simulink model "Final_Project_Part_4_LVLH_kinematics_Template"  (R2022a)
settings: Solver=ode45  StartTime=0.0  StopTime=tspan  RelTol=1e-8  AbsTol=1e-8
model workspace (MATLAB code in the model file):
  | mu = 398601; % km
  | Re = 6378.137; %km
values from neighbouring files (symbols this model uses):
  J = I/12 - m * rx * rx    [aero421_finalProject.m]    (also in aero421_finalProject_D.m)
undefined symbols (not defined in the file or in its folder): E_b_ECI_0, E_b_LVLH_0, q_b_ECI_0, q_b_LVLH_0, r_ECI_0, T_c, v_ECI_0, w_b_ECI_0
settings Model: Creator=emehiel  LastModifiedBy=emehiel
settings SolverCC: AlgebraicLoopSolver=TrustRegion
settings DebuggingCC: UnconnectedInputMsg=warning  UnconnectedOutputMsg=warning  UnconnectedLineMsg=warning  SFMachineParentedDataDiag=warning

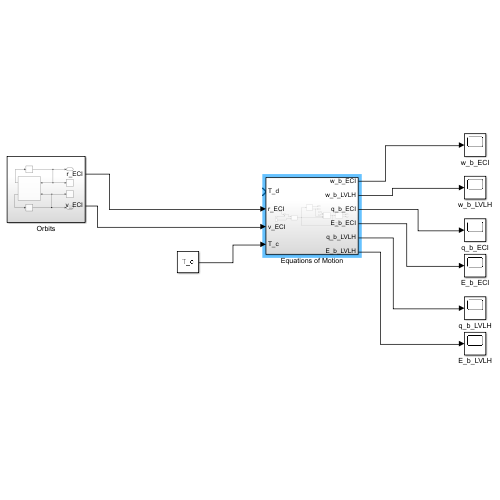
[thumbnail: Simulink's stored preview of the top-level diagram]
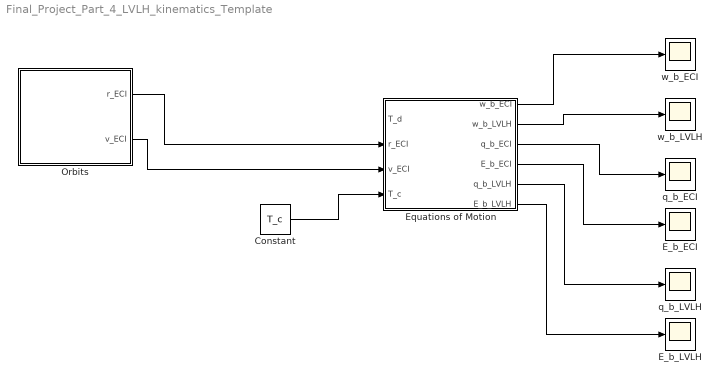
== system Final_Project_Part_4_LVLH_kinematics_Template ==
  Constant : Constant  Value=T_c
  E_b_ECI : Scope
  E_b_LVLH : Scope
  Equations of Motion : Subsystem
  Orbits : Subsystem
  q_b_ECI : Scope
  q_b_LVLH : Scope
  w_b_ECI : Scope
  w_b_LVLH : Scope
  wires:
  Orbits/1(r_ECI) -> Equations of Motion/2(r_ECI)
  Equations of Motion/3(q_b_ECI) -> q_b_ECI/1
  Equations of Motion/1(w_b_ECI) -> w_b_ECI/1
  Equations of Motion/4(E_b_ECI) -> E_b_ECI/1
  Equations of Motion/2(w_b_LVLH) -> w_b_LVLH/1
  Equations of Motion/5(q_b_LVLH) -> q_b_LVLH/1
  Equations of Motion/6(E_b_LVLH) -> E_b_LVLH/1
  Orbits/2(v_ECI) -> Equations of Motion/3(v_ECI)
  Constant/1 -> Equations of Motion/4(T_c)

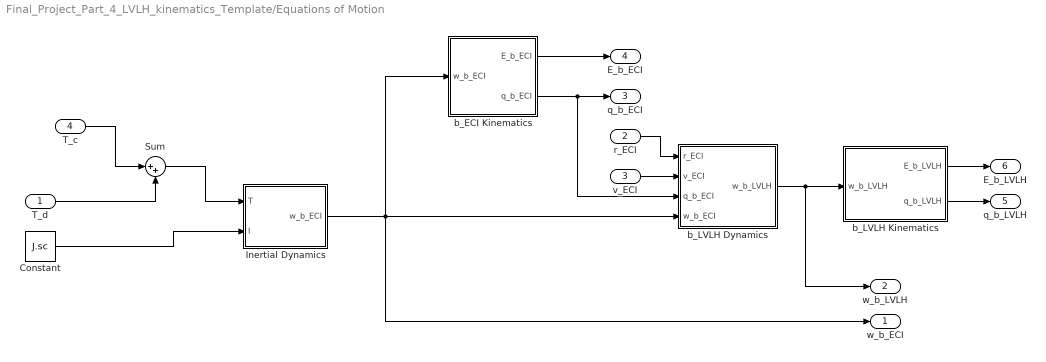
== system Final_Project_Part_4_LVLH_kinematics_Template/Equations of Motion ==
  T_d : Inport
  r_ECI : Inport  Port=2
  v_ECI : Inport  Port=3
  T_c : Inport  Port=4
  Constant : Constant  Value=J.sc
  Inertial Dynamics : Subsystem
  Sum : Sum  Inputs=|++
  b_ECI Kinematics : Subsystem
  b_LVLH Dynamics : Subsystem
  b_LVLH Kinematics : Subsystem
  w_b_ECI : Outport  VectorParamsAs1DForOutWhenUnconnected=off
  w_b_LVLH : Outport  Port=2  PortDimensions=[3 1]  VectorParamsAs1DForOutWhenUnconnected=off
  q_b_ECI : Outport  Port=3  PortDimensions=[4 1]  VectorParamsAs1DForOutWhenUnconnected=off
  E_b_ECI : Outport  Port=4  PortDimensions=[3 1]  VectorParamsAs1DForOutWhenUnconnected=off
  q_b_LVLH : Outport  Port=5  PortDimensions=[4 1]  VectorParamsAs1DForOutWhenUnconnected=off
  E_b_LVLH : Outport  Port=6  PortDimensions=[3 1]  VectorParamsAs1DForOutWhenUnconnected=off
  wires:
  b_ECI Kinematics/1(E_b_ECI) -> E_b_ECI/1
  Constant/1 -> Inertial Dynamics/2(I)
  b_LVLH Kinematics/1(E_b_LVLH) -> E_b_LVLH/1
  Inertial Dynamics/1(w_b_ECI) -> w_b_ECI/1, b_ECI Kinematics/1(w_b_ECI), b_LVLH Dynamics/4(w_b_ECI)
  b_ECI Kinematics/2(q_b_ECI) -> b_LVLH Dynamics/3(q_b_ECI), q_b_ECI/1
  b_LVLH Kinematics/2(q_b_LVLH) -> q_b_LVLH/1
  r_ECI/1 -> b_LVLH Dynamics/1("r_ECI ")
  v_ECI/1 -> b_LVLH Dynamics/2(v_ECI)
  b_LVLH Dynamics/1(w_b_LVLH) -> w_b_LVLH/1, b_LVLH Kinematics/1(w_b_LVLH)
  T_d/1 -> Sum/2
  T_c/1 -> Sum/1
  Sum/1 -> Inertial Dynamics/1(T)

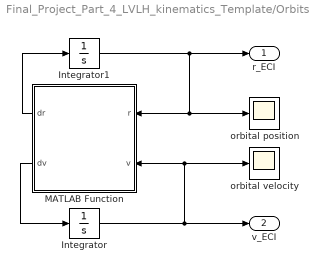
== system Final_Project_Part_4_LVLH_kinematics_Template/Orbits ==
  Integrator : Integrator  InitialCondition=v_ECI_0
  Integrator1 : Integrator  InitialCondition=r_ECI_0
  MATLAB Function : MATLAB Function  TreatAsAtomicUnit=on
  orbital position : Scope
  orbital velocity : Scope
  r_ECI : Outport  VectorParamsAs1DForOutWhenUnconnected=off
  v_ECI : Outport  Port=2  VectorParamsAs1DForOutWhenUnconnected=off
  wires:
  Integrator/1 -> orbital velocity/1, MATLAB Function/2(v), v_ECI/1
  Integrator1/1 -> orbital position/1, MATLAB Function/1(r), r_ECI/1
  MATLAB Function/1(dr) -> Integrator1/1
  MATLAB Function/2(dv) -> Integrator/1

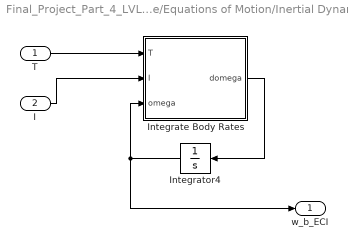
== system Final_Project_Part_4_LVLH_kinematics_Template/Equations of Motion/Inertial Dynamics ==
  T : Inport
  I : Inport  Port=2
  Integrate Body Rates : MATLAB Function  TreatAsAtomicUnit=on
  Integrator4 : Integrator  InitialCondition=w_b_ECI_0
  w_b_ECI : Outport  VectorParamsAs1DForOutWhenUnconnected=off
  wires:
  Integrate Body Rates/1(domega) -> Integrator4/1
  I/1 -> Integrate Body Rates/2(I)
  T/1 -> Integrate Body Rates/1(T)
  Integrator4/1 -> w_b_ECI/1, Integrate Body Rates/3(omega)

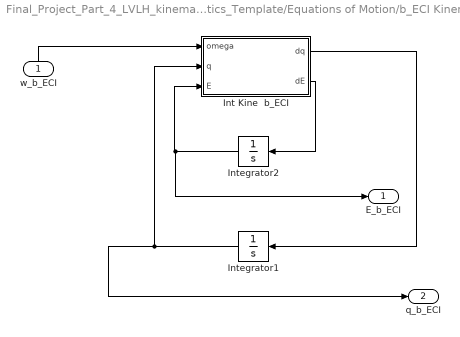
== system Final_Project_Part_4_LVLH_kinematics_Template/Equations of Motion/b_ECI Kinematics ==
  w_b_ECI : Inport
  Int Kine  b_ECI : MATLAB Function  TreatAsAtomicUnit=on
  Integrator1 : Integrator  InitialCondition=q_b_ECI_0
  Integrator2 : Integrator  InitialCondition=E_b_ECI_0
  E_b_ECI : Outport  PortDimensions=[3 1]  VectorParamsAs1DForOutWhenUnconnected=off
  q_b_ECI : Outport  Port=2  PortDimensions=[4 1]  VectorParamsAs1DForOutWhenUnconnected=off
  wires:
  w_b_ECI/1 -> Int Kine  b_ECI/1(omega)
  Int Kine  b_ECI/1(dq) -> Integrator1/1
  Int Kine  b_ECI/2(dE) -> Integrator2/1
  Integrator1/1 -> q_b_ECI/1, Int Kine  b_ECI/2(q)
  Integrator2/1 -> E_b_ECI/1, Int Kine  b_ECI/3(E)

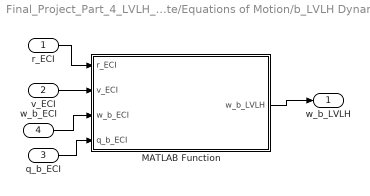
== system Final_Project_Part_4_LVLH_kinematics_Template/Equations of Motion/b_LVLH Dynamics ==
  "r_ECI " : Inport
  v_ECI : Inport  Port=2
  q_b_ECI : Inport  Port=3
  w_b_ECI : Inport  Port=4
  MATLAB Function : MATLAB Function  TreatAsAtomicUnit=on
  w_b_LVLH : Outport  VectorParamsAs1DForOutWhenUnconnected=off
  wires:
  MATLAB Function/1(w_b_LVLH) -> w_b_LVLH/1
  "r_ECI "/1 -> MATLAB Function/1(r_ECI)
  v_ECI/1 -> MATLAB Function/2(v_ECI)
  q_b_ECI/1 -> MATLAB Function/4(q_b_ECI)
  w_b_ECI/1 -> MATLAB Function/3(w_b_ECI)

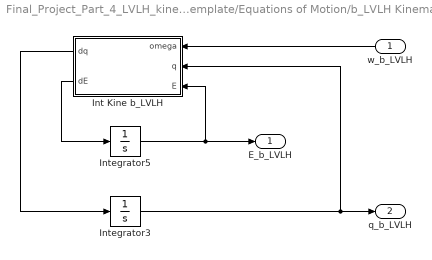
== system Final_Project_Part_4_LVLH_kinematics_Template/Equations of Motion/b_LVLH Kinematics ==
  w_b_LVLH : Inport
  Int Kine b_LVLH : MATLAB Function  TreatAsAtomicUnit=on
  Integrator3 : Integrator  InitialCondition=q_b_LVLH_0
  Integrator5 : Integrator  InitialCondition=E_b_LVLH_0
  E_b_LVLH : Outport  PortDimensions=[3 1]  VectorParamsAs1DForOutWhenUnconnected=off
  q_b_LVLH : Outport  Port=2  VectorParamsAs1DForOutWhenUnconnected=off
  wires:
  Int Kine b_LVLH/1(dq) -> Integrator3/1
  Integrator3/1 -> Int Kine b_LVLH/2(q), q_b_LVLH/1
  Int Kine b_LVLH/2(dE) -> Integrator5/1
  Integrator5/1 -> E_b_LVLH/1, Int Kine b_LVLH/3(E)
  w_b_LVLH/1 -> Int Kine b_LVLH/1(omega)

== matlab function Final_Project_Part_4_LVLH_kinematics_Template/Equations of Motion/Inertial Dynamics/Integrate Body Rates ==
  data: T input; I input; omega input; domega output
function domega = dynamics(T, I, omega)
%#codegen

domega = I\(T - cross(omega, I*omega));

== matlab function Final_Project_Part_4_LVLH_kinematics_Template/Equations of Motion/b_ECI Kinematics/Int Kine  b_ECI ==
  data: omega input; q input; dq output; E input; dE output
function [dq,dE] = kinematics(omega, q, E)
%#codegen

% unpack quaternion

epsilon = q(1:3,1);
eta = q(4,1);

depsilon = 1/2*(eta*eye(3) + vect2cross(epsilon))*omega;
deta = -1/2*epsilon'*omega;

dq = [depsilon; deta];

LBI = 1/cos(E(2))*[cos(E(2)) sin(E(1))*sin(E(2))  cos(E(1))*sin(E(2));
                   0         cos(E(1))*cos(E(2)) -sin(E(1))*cos(E(2));
                   0         sin(E(1))            cos(E(1))];

dE = LBI*omega;

== matlab function Final_Project_Part_4_LVLH_kinematics_Template/Orbits/MATLAB Function ==
  data: r input; dr output; v input; dv output
function [dr,dv] = orbitalDynamics(r, v)
%#codegen

mu = 398601; % km^3/s^2

dr = v;
dv = -mu*r/norm(r)^3;

== matlab function Final_Project_Part_4_LVLH_kinematics_Template/Equations of Motion/b_LVLH Dynamics/MATLAB Function ==
  data: r_ECI input; v_ECI input; w_b_ECI input; q_b_ECI input; w_b_LVLH output
function w_b_LVLH = fcn(r_ECI, v_ECI, w_b_ECI, q_b_ECI)
%#codegen

% Compute the angular velocity of LVLH wrt ECI in Body components

== matlab function Final_Project_Part_4_LVLH_kinematics_Template/Equations of Motion/b_LVLH Kinematics/Int Kine b_LVLH ==
  data: omega input; q input; dq output; E input; dE output
function [dq,dE] = kinematics(omega, q, E)
%#codegen

% unpack quaternion

% compute the derivative of the quaternion components here

% compute the derivative of the Euler Angle components here
